simulink model "Ghost_f4"  (Simulink 8.1)
settings: Solver=ode1  StartTime=0.0  StopTime=inf  FixedStep=Ts  MaxStep=1e-3  RelTol=1e-3
PostLoadFcn:
  | NREL_Mode=3; Ghost_init;
InitFcn:
  | NREL_Mode=3; Ghost_init;
undefined symbols (not defined in the file): F4, Left, Stim, Ts, type, V
libraries: simulink x44, relay_modbus_lib x12, rtio_generic_modbus x6, rtlab x5, cables_lib x3, PHIL_lib x2, breaker_lib x2, power_quality_lib x2, artemis x1, rtio_opalrt_ml605ex1 x1, ssn_lib x1, controllable_grid_lib x1
(part 2 of 2)

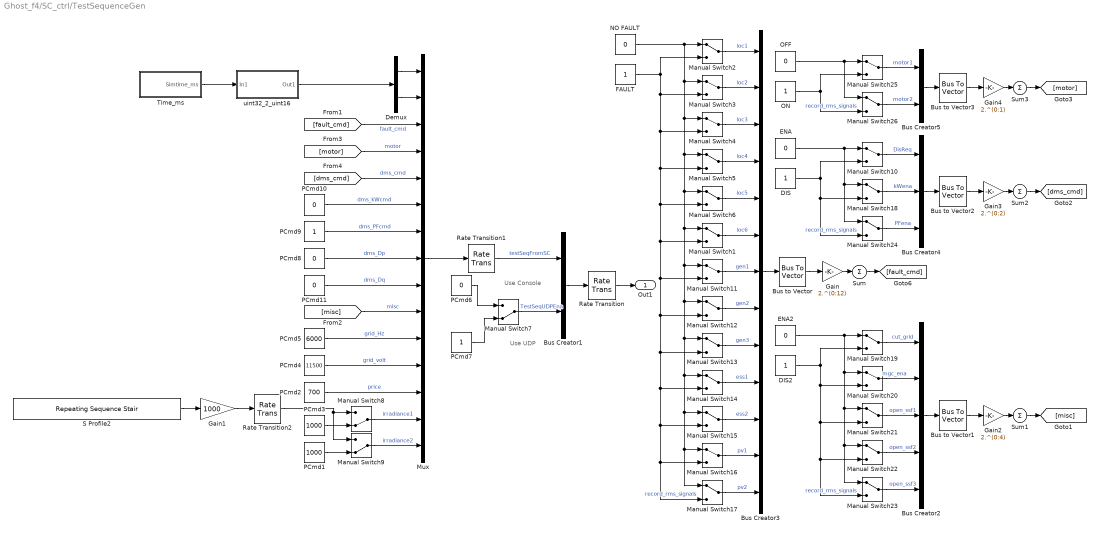
== system Ghost_f4/SC_ctrl/TestSequenceGen ==
  note: Use Console
  note: Use UDP
  Bus Creator1 : BusCreator  Inputs=2
  Bus Creator2 : BusCreator  Inputs=5
  Bus Creator3 : BusCreator  Inputs=13
  Bus Creator4 : BusCreator  Inputs=3
  Bus Creator5 : BusCreator  Inputs=2
  Bus to Vector{,1..3} (4 alike) : BusToVector
  DIS : Constant
  DIS2 : Constant
  Demux : Demux  Outputs=2
  ENA : Constant  Value=0
  ENA2 : Constant  Value=0
  FAULT : Constant
  Gain : Gain  Gain=2.^(0:12)
  Gain1 : Gain  Gain=1000
  Gain2 : Gain  Gain=2.^(0:4)
  Gain3 : Gain  Gain=2.^(0:2)
  Gain4 : Gain  Gain=2.^(0:1)
  Manual Switch{1..6,10..26} (23 alike) : ManualSwitch
  Manual Switch7 : ManualSwitch  CurrentSetting=0
  Manual Switch8 : ManualSwitch  CurrentSetting=0
  Manual Switch9 : ManualSwitch  CurrentSetting=0
  Mux : Mux  Inputs=15
  NO FAULT : Constant  Value=0
  OFF : Constant  Value=0
  ON : Constant
  PCmd1 : Constant  Value=1000
  PCmd10 : Constant  Value=0
  PCmd11 : Constant  Value=0
  PCmd2 : Constant  Value=700
  PCmd3 : Constant  Value=1000
  PCmd4 : Constant  Value=11500
  PCmd5 : Constant  Value=6000
  PCmd6 : Constant  Value=0  SampleTime=[Stim.Ts Ts]
  PCmd7 : Constant
  PCmd8 : Constant  Value=0
  PCmd9 : Constant
  Rate Transition : RateTransition  Deterministic=off
  Rate Transition1 : RateTransition  Deterministic=off  OutPortSampleTime=1e-2
  Rate Transition2 : RateTransition  Deterministic=off  OutPortSampleTime=1e-2
  S Profile2 : simulink/Sources/Repeating Sequence Stair  OutValues=Stim.PV2.Irradiance  tsamp=[Stim.Ts Ts]  OutMin=[]  OutMax=[]  OutDataTypeStr=Inherit: Inherit via back propagation  OutDataType=fixdt(0,8)  ConRadixGroup=Best Precision: Vector-wise  OutScaling=2^-12
  Sum{,1..3} (4 alike) : Sum  Inputs=+
  Time_ms : Subsystem
  uint32_2_uint16 : Subsystem
      mask Display: disp('uint32_2_uint16');
  Out1 : Outport
  wires:
  Manual Switch4/1 -> Bus Creator3/3  "loc3"
  Manual Switch5/1 -> Bus Creator3/4  "loc4"
  [fault_cmd] -> Mux/3  "fault_cmd"
  Bus Creator3/1 -> Bus to Vector/1
  Manual Switch2/1 -> Bus Creator3/1  "loc1"
  Manual Switch6/1 -> Bus Creator3/5  "loc5"
  Manual Switch3/1 -> Bus Creator3/2  "loc2"
  Manual Switch1/1 -> Bus Creator3/6  "loc6"
  Manual Switch13/1 -> Bus Creator3/9  "gen3"
  Manual Switch14/1 -> Bus Creator3/10  "ess1"
  Manual Switch11/1 -> Bus Creator3/7  "gen1"
  Manual Switch15/1 -> Bus Creator3/11  "ess2"
  Manual Switch12/1 -> Bus Creator3/8  "gen2"
  FAULT/1 -> Manual Switch2/2, Manual Switch1/2, Manual Switch12/2, Manual Switch13/2, Manual Switch14/2, Manual Switch17/2, Manual Switch16/2, Manual Switch15/2, Manual Switch11/2, Manual Switch6/2, Manual Switch5/2, Manual Switch4/2, Manual Switch3/2  "record_rms_signals"
  NO FAULT/1 -> Manual Switch12/1, Manual Switch13/1, Manual Switch14/1, Manual Switch15/1, Manual Switch17/1, Manual Switch16/1, Manual Switch11/1, Manual Switch1/1, Manual Switch6/1, Manual Switch5/1, Manual Switch4/1, Manual Switch3/1, Manual Switch2/1
  Manual Switch16/1 -> Bus Creator3/12  "pv1"
  Manual Switch17/1 -> Bus Creator3/13  "pv2"
  Bus to Vector/1 -> Gain/1
  Gain/1 -> Sum/1
  Sum/1 -> [fault_cmd]
  Mux/1 -> Rate Transition1/1
  Bus Creator1/1 -> Rate Transition/1
  Manual Switch7/1 -> Bus Creator1/2  "TestSeqUDPEna"
  PCmd6/1 -> Manual Switch7/1
  PCmd7/1 -> Manual Switch7/2
  Rate Transition/1 -> Out1/1
  PCmd3/1 -> Manual Switch8/2
  Manual Switch9/1 -> Mux/15  "irradiance2"
  PCmd1/1 -> Manual Switch9/2
  Manual Switch8/1 -> Mux/14  "irradiance1"
  PCmd2/1 -> Mux/13  "price"
  Gain1/1 -> Rate Transition2/1
  Time_ms/1(Simtime_ms) -> uint32_2_uint16/1(In1)
  Demux/1 -> Mux/1
  Demux/2 -> Mux/2
  PCmd4/1 -> Mux/12  "grid_volt"
  PCmd5/1 -> Mux/11  "grid_Hz"
  [misc] -> Mux/10  "misc"
  [motor] -> Mux/4  "motor"
  [dms_cmd] -> Mux/5  "dms_cmd"
  PCmd8/1 -> Mux/8  "dms_Dp"
  PCmd9/1 -> Mux/7  "dms_PFcmd"
  PCmd10/1 -> Mux/6  "dms_kWcmd"
  PCmd11/1 -> Mux/9  "dms_Dq"
  Manual Switch21/1 -> Bus Creator2/3  "open_ssf1"
  Manual Switch22/1 -> Bus Creator2/4  "open_ssf2"
  Bus Creator2/1 -> Bus to Vector1/1
  Manual Switch19/1 -> Bus Creator2/1  "cut_grid"
  Manual Switch23/1 -> Bus Creator2/5  "open_ssf3"
  Manual Switch20/1 -> Bus Creator2/2  "mgc_ena"
  DIS2/1 -> Manual Switch20/2, Manual Switch21/2, Manual Switch22/2, Manual Switch23/2, Manual Switch19/2  "record_rms_signals"
  ENA2/1 -> Manual Switch19/1, Manual Switch20/1, Manual Switch21/1, Manual Switch22/1, Manual Switch23/1
  Bus to Vector1/1 -> Gain2/1
  Gain2/1 -> Sum1/1
  Sum1/1 -> [misc]
  Manual Switch24/1 -> Bus Creator4/3  "PFena"
  Bus Creator4/1 -> Bus to Vector2/1
  Manual Switch10/1 -> Bus Creator4/1  "DisReq"
  Manual Switch18/1 -> Bus Creator4/2  "kWena"
  DIS/1 -> Manual Switch10/2, Manual Switch24/2, Manual Switch18/2  "record_rms_signals"
  ENA/1 -> Manual Switch24/1, Manual Switch18/1, Manual Switch10/1
  Bus to Vector2/1 -> Gain3/1
  Gain3/1 -> Sum2/1
  Sum2/1 -> [dms_cmd]
  Bus Creator5/1 -> Bus to Vector3/1
  Manual Switch25/1 -> Bus Creator5/1  "motor1"
  Manual Switch26/1 -> Bus Creator5/2  "motor2"
  ON/1 -> Manual Switch26/2, Manual Switch25/2  "record_rms_signals"
  OFF/1 -> Manual Switch25/1, Manual Switch26/1
  Bus to Vector3/1 -> Gain4/1
  Gain4/1 -> Sum3/1
  Sum3/1 -> [motor]
  S Profile2/1 -> Gain1/1
  uint32_2_uint16/1(Out1) -> Demux/1
  Rate Transition1/1 -> Bus Creator1/1  "testSeqFromSC"
  Rate Transition2/1 -> Manual Switch9/1, Manual Switch8/1

== system Ghost_f4/SS_F4_RELAY_HOUSING/BESS_data ==
  note: 0 .... 10000
      | 0 ... 100%
  Bus Selector1 : BusSelector  OutputSignals=Battery.SoC
  Bus Selector9 : BusSelector  OutputSignals=ESS_DATA
  Constant2 : Constant  Value=0
  Mux : Mux  Inputs=2
  Scale_SoC : Gain  Gain=100
  Out1 : Outport
  wires:
  Scale_SoC/1 -> Out1/1
  [F4_MS_IN] -> Bus Selector9/1
  Bus Selector9/1 -> Bus Selector1/1  "<ESS_DATA>"
  Bus Selector1/1 -> Mux/2  "<SoC>"
  Constant2/1 -> Mux/1
  Mux/1 -> Scale_SoC/1

== system Ghost_f4/SS_F4_RELAY_HOUSING/DieselData ==
  Bus Selector : BusSelector  OutputSignals=GEN3_DATA.gen.gal_per_hr,GEN3_DATA.cb.relay_out.m.Vpu
  Constant1 : Constant  Value=0
  Constant4 : Constant  Value=0
  Mux : Mux
  scale_diesel1 : Gain  Gain=100
  scale_diesel2 : Gain  Gain=100
  Out2 : Outport
  wires:
  [F4_MS_IN] -> Bus Selector/1
  Bus Selector/1 -> scale_diesel1/1  "<gal_per_hr>"
  scale_diesel1/1 -> Mux/2
  Constant4/1 -> Mux/1
  Mux/1 -> Out2/1
  scale_diesel2/1 -> Mux/4
  Bus Selector/2 -> scale_diesel2/1  "<Vpu>"
  Constant1/1 -> Mux/3

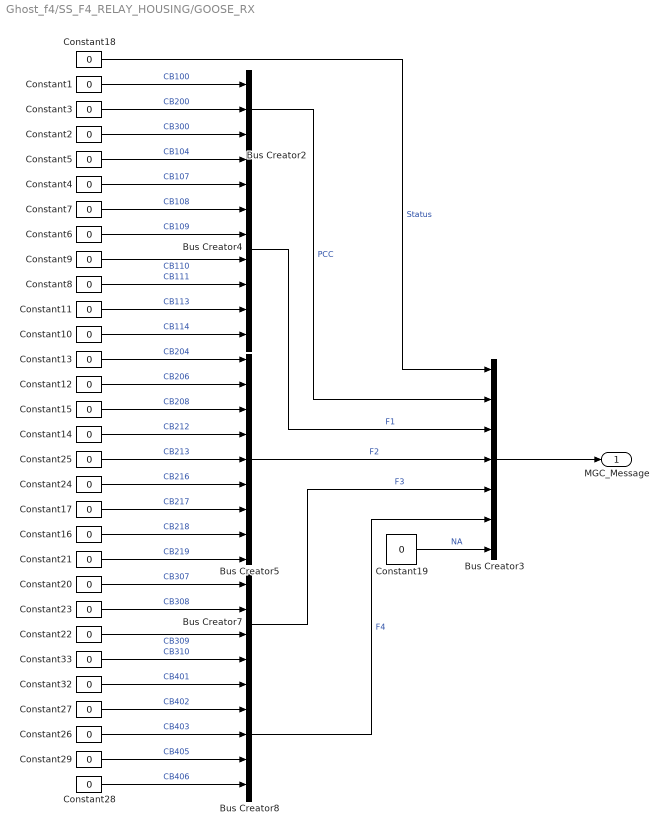
== system Ghost_f4/SS_F4_RELAY_HOUSING/GOOSE_RX  ==
  Bus Creator2 : BusCreator  Inputs=3
  Bus Creator3 : BusCreator  Inputs=7
  Bus Creator4 : BusCreator  Inputs=8
  Bus Creator5 : BusCreator  Inputs=9
  Bus Creator7 : BusCreator
  Bus Creator8 : BusCreator  Inputs=5
  Constant{1..29,32..33} (31 alike) : Constant  Value=0
  MGC_Message : Outport
  wires:
  Constant18/1 -> Bus Creator3/1  "Status"
  Bus Creator3/1 -> MGC_Message/1
  Constant1/1 -> Bus Creator2/1  "CB100"
  Constant3/1 -> Bus Creator2/2  "CB200"
  Constant2/1 -> Bus Creator2/3  "CB300"
  Bus Creator2/1 -> Bus Creator3/2  "PCC"
  Constant7/1 -> Bus Creator4/3  "CB108"
  Constant6/1 -> Bus Creator4/4  "CB109"
  Constant4/1 -> Bus Creator4/2  "CB107"
  Constant9/1 -> Bus Creator4/5  "CB110"
  Constant5/1 -> Bus Creator4/1  "CB104"
  Constant8/1 -> Bus Creator4/6  "CB111"
  Constant11/1 -> Bus Creator4/7  "CB113"
  Constant10/1 -> Bus Creator4/8  "CB114"
  Bus Creator4/1 -> Bus Creator3/3  "F1"
  Constant21/1 -> Bus Creator5/9  "CB219"
  Constant24/1 -> Bus Creator5/6  "CB216"
  Constant17/1 -> Bus Creator5/7  "CB217"
  Constant25/1 -> Bus Creator5/5  "CB213"
  Constant16/1 -> Bus Creator5/8  "CB218"
  Constant15/1 -> Bus Creator5/3  "CB208"
  Constant13/1 -> Bus Creator5/1  "CB204"
  Constant14/1 -> Bus Creator5/4  "CB212"
  Constant12/1 -> Bus Creator5/2  "CB206"
  Bus Creator5/1 -> Bus Creator3/4  "F2"
  Bus Creator8/1 -> Bus Creator3/6  "F4"
  Constant28/1 -> Bus Creator8/5  "CB406"
  Constant26/1 -> Bus Creator8/3  "CB403"
  Bus Creator7/1 -> Bus Creator3/5  "F3"
  Constant33/1 -> Bus Creator7/4  "CB310"
  Constant22/1 -> Bus Creator7/3  "CB309"
  Constant23/1 -> Bus Creator7/2  "CB308"
  Constant20/1 -> Bus Creator7/1  "CB307"
  Constant19/1 -> Bus Creator3/7  "NA"
  Constant29/1 -> Bus Creator8/4  "CB405"
  Constant27/1 -> Bus Creator8/2  "CB402"
  Constant32/1 -> Bus Creator8/1  "CB401"

== system Ghost_f4/SS_F4_RELAY_HOUSING/MGC_controller ==
  Bus Selector1 : BusSelector  OutputSignals=GEN3_DATA,ESS_DATA,PV_DATA
  Bus Selector2 : BusSelector  OutputSignals=ctrl.raw
  Bus Selector3 : BusSelector  OutputSignals=raw
  Bus Selector4 : BusSelector  OutputSignals=raw
  Bus Selector5 : BusSelector  OutputSignals=F4_CB_CTRL  OutputAsBus=on
  Bus to Vector : BusToVector
  Constant : Constant  Value=zeros(1,14)
  Constant1 : Constant  Value=zeros(1,19)
  Constant2 : Constant  Value=zeros(1,10)
  Constant3 : Constant  Value=zeros(1,3)
  Constant{4..7} (4 alike) : Constant  Value=zeros(1,8)
  Vector Concatenate : Concatenate  NumInputs=12
  MGC_controller : Outport
  wires:
  Bus Selector4/1 -> Vector Concatenate/12  "<raw>"
  Constant7/1 -> Vector Concatenate/9
  Constant6/1 -> Vector Concatenate/8
  Constant5/1 -> Vector Concatenate/7
  Constant4/1 -> Vector Concatenate/6
  Bus Selector2/1 -> Vector Concatenate/10  "<raw>"
  Bus Selector3/1 -> Vector Concatenate/11  "<raw>"
  Bus Selector1/3 -> Bus Selector4/1  "<PV_DATA>"
  Bus Selector1/2 -> Bus Selector3/1  "<ESS_DATA>"
  Bus Selector1/1 -> Bus Selector2/1  "<GEN3_DATA>"
  [F4_MS_IN] -> Bus Selector1/1
  Constant2/1 -> Vector Concatenate/3
  Constant1/1 -> Vector Concatenate/2
  Constant/1 -> Vector Concatenate/1
  Constant3/1 -> Vector Concatenate/5
  Vector Concatenate/1 -> MGC_controller/1
  Bus to Vector/1 -> Vector Concatenate/4
  [F4_RELAY_OUT] -> Bus Selector5/1
  Bus Selector5/1 -> Bus to Vector/1

== system Ghost_f4/SS_F4_RELAY_HOUSING/Misc_data ==
  note: Data ordered as:
      | I-P-C
      | kW-VRMSLL
  Bus Creator : BusCreator  Inputs=2
  Constant : Constant  Value=0
  Constant1 : Constant  Value=zeros(1,9)
  Mux8 : Mux  Inputs=2
  Mux9 : Mux  Inputs=2
  VRMSLL : Subsystem
  kW : Subsystem
  scale_load : Gain
  Out1 : Outport
  wires:
  scale_load/1 -> Mux9/1
  [F4_MS_IN] -> Bus Creator/1  "F4"
  Bus Creator/1 -> VRMSLL/1(In1), kW/1(In1)
  Mux8/1 -> scale_load/1
  Constant1/1 -> Mux9/2
  Mux9/1 -> Out1/1
  Constant/1 -> Bus Creator/2  "zero"
  kW/1(Out1) -> Mux8/1
  VRMSLL/1(Out1) -> Mux8/2

== system Ghost_f4/SS_F4_RELAY_HOUSING/Power_quality_data ==
  Rst : Inport
  Bus Selector2 : BusSelector  OutputSignals=F4_CB_1.m.Vpu,F4_CB_2.m.Vpu,F4_CB_5.m.Vpu  OutputAsBus=on
  Bus Selector7 : BusSelector  OutputSignals=F4_CB_1.m.Hz,F4_CB_2.m.Hz,F4_CB_5.m.Hz  OutputAsBus=on
  Bus to Vector : BusToVector
  Bus to Vector3 : BusToVector
  Constant3 : Constant  Value=zeros(1,20)
  Constant4 : Constant  Value=zeros(1,20)
  IEEE1547a_Hz : power_quality_lib/IEEE1547a_Hz
  IEEE1547a_Volt : power_quality_lib/IEEE1547a_Hz
  Mux : Mux  Inputs=2
  Mux2 : Mux  Inputs=2
  Mux3 : Mux  Inputs=2
  Out1 : Outport
  wires:
  Bus to Vector3/1 -> IEEE1547a_Volt/1
  Bus Selector2/1 -> Bus to Vector3/1
  [F4_RELAY_OUT] -> Bus Selector7/1
  [F4_RELAY_OUT] -> Bus Selector2/1
  Constant3/1 -> Mux/1
  Bus to Vector/1 -> IEEE1547a_Hz/1
  Mux/1 -> Mux3/1
  Mux2/1 -> Mux3/2
  IEEE1547a_Volt/1 -> Mux2/2
  Mux3/1 -> Out1/1
  Constant4/1 -> Mux2/1
  Bus Selector7/1 -> Bus to Vector/1
  IEEE1547a_Hz/1 -> Mux/2
  Rst/1 -> IEEE1547a_Volt/2, IEEE1547a_Hz/2

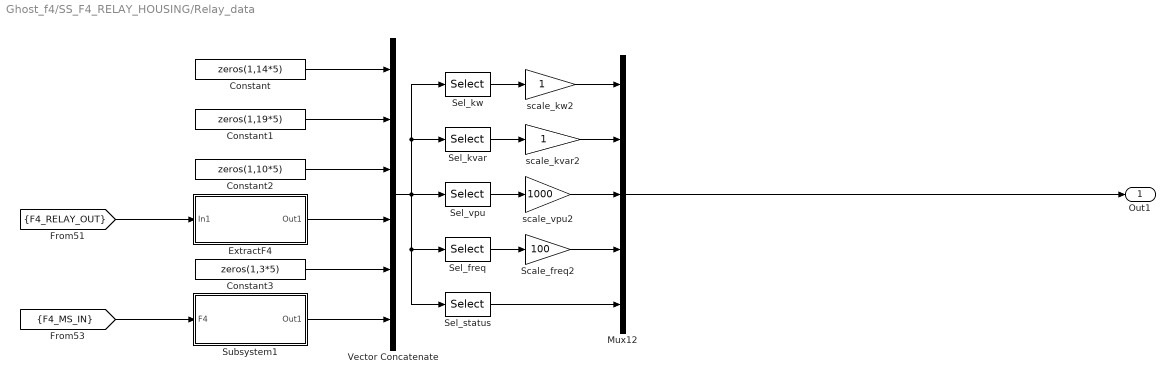
== system Ghost_f4/SS_F4_RELAY_HOUSING/Relay_data ==
  Constant : Constant  Value=zeros(1,14*5)
  Constant1 : Constant  Value=zeros(1,19*5)
  Constant2 : Constant  Value=zeros(1,10*5)
  Constant3 : Constant  Value=zeros(1,3*5)
  ExtractF4 : Subsystem
      mask Display: disp('Generic F4 relays\nID = 44 .. 49')
  Mux12 : Mux  Inputs=5
  Scale_freq2 : Gain  Gain=100
  Sel_freq : Selector  InputPortWidth=59*5  IndexOptions=Index vector (dialog)  Indices=[4:5:59*5]  OutputSizes=1
  Sel_kvar : Selector  InputPortWidth=59*5  IndexOptions=Index vector (dialog)  Indices=[2:5:59*5]  OutputSizes=1
  Sel_kw : Selector  InputPortWidth=59*5  IndexOptions=Index vector (dialog)  Indices=[1:5:59*5]  OutputSizes=1
  Sel_status : Selector  InputPortWidth=59*5  IndexOptions=Index vector (dialog)  Indices=[5:5:59*5]  OutputSizes=1
  Sel_vpu : Selector  InputPortWidth=59*5  IndexOptions=Index vector (dialog)  Indices=[3:5:59*5]  OutputSizes=1
  Subsystem1 : Subsystem
      mask Display: disp('GEN1,ESS1,PV1\nGEN2,GEN3,ESS2,PV1\nID = 53 .. 59')
  Vector Concatenate : Concatenate  NumInputs=6
  scale_kvar2 : Gain
  scale_kw2 : Gain
  scale_vpu2 : Gain  Gain=1000
  Out1 : Outport
  wires:
  [F4_RELAY_OUT] -> ExtractF4/1(In1)
  ExtractF4/1(Out1) -> Vector Concatenate/4
  Constant2/1 -> Vector Concatenate/3
  Constant1/1 -> Vector Concatenate/2
  Constant/1 -> Vector Concatenate/1
  Constant3/1 -> Vector Concatenate/5
  [F4_MS_IN] -> Subsystem1/1(F4)
  Subsystem1/1(Out1) -> Vector Concatenate/6
  Mux12/1 -> Out1/1
  scale_kw2/1 -> Mux12/1
  scale_kvar2/1 -> Mux12/2
  Scale_freq2/1 -> Mux12/4
  scale_vpu2/1 -> Mux12/3
  Sel_kw/1 -> scale_kw2/1
  Sel_status/1 -> Mux12/5
  Sel_freq/1 -> Scale_freq2/1
  Sel_vpu/1 -> scale_vpu2/1
  Sel_kvar/1 -> scale_kvar2/1
  Vector Concatenate/1 -> Sel_status/1, Sel_freq/1, Sel_vpu/1, Sel_kvar/1, Sel_kw/1

== system Ghost_f4/SS_F4_RELAY_HOUSING/Time_ms ==
  Constant4 : Constant  Value=Ts/1e-3
  Sum : Sum  Inputs=++|
  Unit Delay : UnitDelay  SampleTime=-1
  Simtime_ms : Outport
  wires:
  Sum/1 -> Simtime_ms/1, Unit Delay/1
  Constant4/1 -> Sum/2
  Unit Delay/1 -> Sum/1

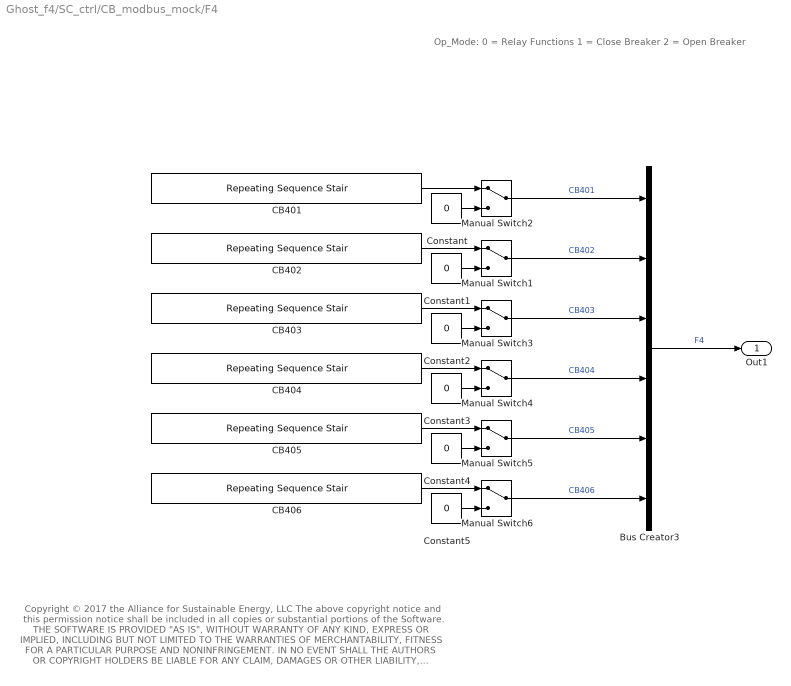
== system Ghost_f4/SC_ctrl/CB_modbus_mock/F4 ==
  note: Op_Mode:
      | 0 = Relay Functions
      | 1 = Close Breaker
      | 2 = Open Breaker
  note: Copyright © 2017 the Alliance for Sustainable Energy, LLC
      |
      | The above copyright notice and this permission notice shall be included in all copies or substantial portions of the Software.
      |
      | THE SOFTWARE IS PROVIDED "AS IS", WITHOUT WARRANTY OF ANY KIND, EXPRESS OR IMPLIED, INCLUDING
      | BUT NOT LIMITED TO THE WARRANTIES OF MERCHANTABILITY, FITNESS FOR A PARTICULAR PURPOSE AND
      | NONINFRINGEMENT. IN NO EVENT SHALL THE AUTHORS OR COPYRIGHT HOLDERS BE LIABLE FOR ANY CLAIM,
      |  DAMAGES OR OTHER LIABILITY, WHETHER IN AN ACTION OF CONTRACT, TORT OR OTHERWISE, ARISING FROM,
      | OUT OF OR IN CONNECTION WITH THE SOFTWARE OR THE USE OR OTHER DEALINGS IN THE SOFTWARE
  Bus Creator3 : BusCreator  Inputs=6
  CB401 : simulink/Sources/Repeating Sequence Stair  OutValues=Stim.CB.CB401  tsamp=[Stim.Ts Ts]  OutMin=[]  OutMax=[]  OutDataTypeStr=Inherit: Inherit via back propagation  OutDataType=fixdt(0,8)  ConRadixGroup=Best Precision: Vector-wise  OutScaling=2^-12
  CB402 : simulink/Sources/Repeating Sequence Stair  OutValues=Stim.CB.CB402  tsamp=[Stim.Ts Ts]  OutMin=[]  OutMax=[]  OutDataTypeStr=Inherit: Inherit via back propagation  OutDataType=fixdt(0,8)  ConRadixGroup=Best Precision: Vector-wise  OutScaling=2^-12
  CB403 : simulink/Sources/Repeating Sequence Stair  OutValues=Stim.CB.CB403  tsamp=[Stim.Ts Ts]  OutMin=[]  OutMax=[]  OutDataTypeStr=Inherit: Inherit via back propagation  OutDataType=fixdt(0,8)  ConRadixGroup=Best Precision: Vector-wise  OutScaling=2^-12
  CB404 : simulink/Sources/Repeating Sequence Stair  OutValues=Stim.CB.CB404  tsamp=[Stim.Ts Ts]  OutMin=[]  OutMax=[]  OutDataTypeStr=Inherit: Inherit via back propagation  OutDataType=fixdt(0,8)  ConRadixGroup=Best Precision: Vector-wise  OutScaling=2^-12
  CB405 : simulink/Sources/Repeating Sequence Stair  OutValues=Stim.CB.CB405  tsamp=[Stim.Ts Ts]  OutMin=[]  OutMax=[]  OutDataTypeStr=Inherit: Inherit via back propagation  OutDataType=fixdt(0,8)  ConRadixGroup=Best Precision: Vector-wise  OutScaling=2^-12
  CB406 : simulink/Sources/Repeating Sequence Stair  OutValues=Stim.CB.CB406  tsamp=[Stim.Ts Ts]  OutMin=[]  OutMax=[]  OutDataTypeStr=Inherit: Inherit via back propagation  OutDataType=fixdt(0,8)  ConRadixGroup=Best Precision: Vector-wise  OutScaling=2^-12
  Constant{,1..5} (6 alike) : Constant  Value=0
  Manual Switch{1..6} (6 alike) : ManualSwitch
  Out1 : Outport
  wires:
  Bus Creator3/1 -> Out1/1  "F4"
  CB401/1 -> Manual Switch2/1
  Constant/1 -> Manual Switch2/2
  Manual Switch2/1 -> Bus Creator3/1  "CB401"
  Manual Switch6/1 -> Bus Creator3/6  "CB406"
  CB402/1 -> Manual Switch1/1
  Manual Switch1/1 -> Bus Creator3/2  "CB402"
  Manual Switch5/1 -> Bus Creator3/5  "CB405"
  Manual Switch3/1 -> Bus Creator3/3  "CB403"
  Manual Switch4/1 -> Bus Creator3/4  "CB404"
  Constant1/1 -> Manual Switch1/2
  CB403/1 -> Manual Switch3/1
  Constant2/1 -> Manual Switch3/2
  CB404/1 -> Manual Switch4/1
  Constant3/1 -> Manual Switch4/2
  CB405/1 -> Manual Switch5/1
  Constant4/1 -> Manual Switch5/2
  CB406/1 -> Manual Switch6/1
  Constant5/1 -> Manual Switch6/2

== system Ghost_f4/SC_ctrl/ESS2 control/Tuning ==
  note: Not applicable
      | for PV
  Bus Creator : BusCreator  Inputs=7
  Constant : Constant  Value=2  SampleTime=[Stim.Ts Ts]
  Constant1 : Constant  Value=0.6e-3  SampleTime=[Stim.Ts Ts]
  Constant10 : Constant  Value=0  SampleTime=[Stim.Ts Ts]
  Constant2 : Constant  Value=180  SampleTime=[Stim.Ts Ts]
  Constant3 : Constant  Value=3200  SampleTime=[Stim.Ts Ts]
  Constant4 : Constant  SampleTime=[Stim.Ts Ts]
  Constant9 : Constant  SampleTime=[Stim.Ts Ts]
  Tuning : Outport
  wires:
  Bus Creator/1 -> Tuning/1
  Constant/1 -> Bus Creator/1  "csi_kp"
  Constant1/1 -> Bus Creator/2  "csi_Ti"
  Constant2/1 -> Bus Creator/3  "pll_kp"
  Constant3/1 -> Bus Creator/4  "pll_ki"
  Constant4/1 -> Bus Creator/5  "vff_ena"
  Constant10/1 -> Bus Creator/7  "batt_soc_rst"
  Constant9/1 -> Bus Creator/6  "batt_cap_div"

== system Ghost_f4/SC_ctrl/PV2 control/Tuning ==
  note: Not applicable
      | for PV
  note: Nominal Insulation = 1000W/m^2
  note: A
      | --------
      | W/m^2
  Bus Creator : BusCreator  Inputs=13
  Constant : Constant  Value=2  SampleTime=[Stim.Ts Ts]
  Constant1 : Constant  Value=0.6e-3  SampleTime=[Stim.Ts Ts]
  Constant10 : Constant  SampleTime=[Stim.Ts Ts]
  Constant12 : Constant  Value=0.2
  Constant13 : Constant  Value=0
  Constant2 : Constant  Value=180  SampleTime=[Stim.Ts Ts]
  Constant3 : Constant  Value=3200  SampleTime=[Stim.Ts Ts]
  Constant4 : Constant  SampleTime=[Stim.Ts Ts]
  Constant5 : Constant  Value=31
  Constant6 : Constant  Value=36
  Constant7 : Constant
  Constant8 : Constant  Value=590
  Constant9 : Constant  SampleTime=[Stim.Ts Ts]
  Tuning : Outport
  wires:
  Constant4/1 -> Bus Creator/5  "vff_ena"
  Constant3/1 -> Bus Creator/4  "pll_ki"
  Constant2/1 -> Bus Creator/3  "pll_kp"
  Constant1/1 -> Bus Creator/2  "csi_Ti"
  Constant/1 -> Bus Creator/1  "csi_kp"
  Bus Creator/1 -> Tuning/1
  Constant6/1 -> Bus Creator/7  "ParallelN"
  Constant5/1 -> Bus Creator/6  "SeriesN"
  Constant7/1 -> Bus Creator/8  "Imin"
  Constant8/1 -> Bus Creator/9  "Vref"
  Constant10/1 -> Bus Creator/11  "batt_soc_rst"
  Constant9/1 -> Bus Creator/10  "batt_cap_div"
  Constant13/1 -> Bus Creator/12  "ConstCurEna"
  Constant12/1 -> Bus Creator/13  "ConstCurGain"

== system Ghost_f4/SC_ctrl/Plots/status_bits_extract ==
  In1 : Inport
  Bias : Bias  Bias=[9:-1:0]*1.1
  Data Type Conversion : DataTypeConversion  OutDataTypeStr=uint16
  Data Type Conversion1 : DataTypeConversion  OutDataTypeStr=double
  Extract Bits1 : simulink/Logic and Bit Operations/Extract Bits  bitsToExtract=Range of bits  numBits=8  bitIdxRange=0  outScalingMode=Treat bit field as an integer
  Extract Bits10 : simulink/Logic and Bit Operations/Extract Bits  bitsToExtract=Range of bits  numBits=8  bitIdxRange=9  outScalingMode=Treat bit field as an integer
  Extract Bits2 : simulink/Logic and Bit Operations/Extract Bits  bitsToExtract=Range of bits  numBits=8  bitIdxRange=1  outScalingMode=Treat bit field as an integer
  Extract Bits3 : simulink/Logic and Bit Operations/Extract Bits  bitsToExtract=Range of bits  numBits=8  bitIdxRange=2  outScalingMode=Treat bit field as an integer
  Extract Bits4 : simulink/Logic and Bit Operations/Extract Bits  bitsToExtract=Range of bits  numBits=8  bitIdxRange=3  outScalingMode=Treat bit field as an integer
  Extract Bits5 : simulink/Logic and Bit Operations/Extract Bits  bitsToExtract=Range of bits  numBits=8  bitIdxRange=4  outScalingMode=Treat bit field as an integer
  Extract Bits6 : simulink/Logic and Bit Operations/Extract Bits  bitsToExtract=Range of bits  numBits=8  bitIdxRange=5  outScalingMode=Treat bit field as an integer
  Extract Bits7 : simulink/Logic and Bit Operations/Extract Bits  bitsToExtract=Range of bits  numBits=8  bitIdxRange=6  outScalingMode=Treat bit field as an integer
  Extract Bits8 : simulink/Logic and Bit Operations/Extract Bits  bitsToExtract=Range of bits  numBits=8  bitIdxRange=7  outScalingMode=Treat bit field as an integer
  Extract Bits9 : simulink/Logic and Bit Operations/Extract Bits  bitsToExtract=Range of bits  numBits=8  bitIdxRange=8  outScalingMode=Treat bit field as an integer
  Mux : Mux  Inputs=10
  Out1 : Outport
  wires:
  Bias/1 -> Out1/1
  Extract Bits5/1 -> Mux/5
  In1/1 -> Data Type Conversion/1
  Extract Bits2/1 -> Mux/2
  Data Type Conversion/1 -> Extract Bits1/1, Extract Bits2/1, Extract Bits3/1, Extract Bits4/1, Extract Bits5/1, Extract Bits8/1, Extract Bits10/1, Extract Bits9/1, Extract Bits7/1, Extract Bits6/1
  Mux/1 -> Data Type Conversion1/1
  Extract Bits1/1 -> Mux/1
  Data Type Conversion1/1 -> Bias/1
  Extract Bits10/1 -> Mux/10
  Extract Bits8/1 -> Mux/8
  Extract Bits9/1 -> Mux/9
  Extract Bits3/1 -> Mux/3
  Extract Bits4/1 -> Mux/4
  Extract Bits7/1 -> Mux/7
  Extract Bits6/1 -> Mux/6

== system Ghost_f4/SC_ctrl/Plots/status_bits_extract1 ==
  In1 : Inport
  Bias : Bias  Bias=[9:-1:0]*1.1
  Data Type Conversion : DataTypeConversion  OutDataTypeStr=uint16
  Data Type Conversion1 : DataTypeConversion  OutDataTypeStr=double
  Extract Bits1 : simulink/Logic and Bit Operations/Extract Bits  bitsToExtract=Range of bits  numBits=8  bitIdxRange=0  outScalingMode=Treat bit field as an integer
  Extract Bits10 : simulink/Logic and Bit Operations/Extract Bits  bitsToExtract=Range of bits  numBits=8  bitIdxRange=9  outScalingMode=Treat bit field as an integer
  Extract Bits2 : simulink/Logic and Bit Operations/Extract Bits  bitsToExtract=Range of bits  numBits=8  bitIdxRange=1  outScalingMode=Treat bit field as an integer
  Extract Bits3 : simulink/Logic and Bit Operations/Extract Bits  bitsToExtract=Range of bits  numBits=8  bitIdxRange=2  outScalingMode=Treat bit field as an integer
  Extract Bits4 : simulink/Logic and Bit Operations/Extract Bits  bitsToExtract=Range of bits  numBits=8  bitIdxRange=3  outScalingMode=Treat bit field as an integer
  Extract Bits5 : simulink/Logic and Bit Operations/Extract Bits  bitsToExtract=Range of bits  numBits=8  bitIdxRange=4  outScalingMode=Treat bit field as an integer
  Extract Bits6 : simulink/Logic and Bit Operations/Extract Bits  bitsToExtract=Range of bits  numBits=8  bitIdxRange=5  outScalingMode=Treat bit field as an integer
  Extract Bits7 : simulink/Logic and Bit Operations/Extract Bits  bitsToExtract=Range of bits  numBits=8  bitIdxRange=6  outScalingMode=Treat bit field as an integer
  Extract Bits8 : simulink/Logic and Bit Operations/Extract Bits  bitsToExtract=Range of bits  numBits=8  bitIdxRange=7  outScalingMode=Treat bit field as an integer
  Extract Bits9 : simulink/Logic and Bit Operations/Extract Bits  bitsToExtract=Range of bits  numBits=8  bitIdxRange=8  outScalingMode=Treat bit field as an integer
  Mux : Mux  Inputs=10
  Out1 : Outport
  wires:
  Extract Bits6/1 -> Mux/6
  Extract Bits7/1 -> Mux/7
  Extract Bits4/1 -> Mux/4
  Extract Bits3/1 -> Mux/3
  Extract Bits9/1 -> Mux/9
  Extract Bits8/1 -> Mux/8
  Extract Bits10/1 -> Mux/10
  Data Type Conversion1/1 -> Bias/1
  Extract Bits1/1 -> Mux/1
  Mux/1 -> Data Type Conversion1/1
  Data Type Conversion/1 -> Extract Bits6/1, Extract Bits7/1, Extract Bits9/1, Extract Bits10/1, Extract Bits8/1, Extract Bits5/1, Extract Bits4/1, Extract Bits3/1, Extract Bits2/1, Extract Bits1/1
  Extract Bits2/1 -> Mux/2
  In1/1 -> Data Type Conversion/1
  Extract Bits5/1 -> Mux/5
  Bias/1 -> Out1/1

== system Ghost_f4/SC_ctrl/TestSequenceGen/Time_ms ==
  Constant4 : Constant  Value=10
  Sum : Sum  Inputs=++|
  Unit Delay : UnitDelay  SampleTime=1e-2
  Simtime_ms : Outport
  wires:
  Unit Delay/1 -> Sum/1
  Constant4/1 -> Sum/2
  Sum/1 -> Unit Delay/1, Simtime_ms/1

== system Ghost_f4/SC_ctrl/TestSequenceGen/uint32_2_uint16 ==
  In1 : Inport
  Data Type Conversion : DataTypeConversion  OutDataTypeStr=uint32
  Data Type Conversion1 : DataTypeConversion  OutDataTypeStr=double
  Data Type Conversion2 : DataTypeConversion  OutDataTypeStr=double
  Extract Bits : simulink/Logic and Bit Operations/Extract Bits  bitsToExtract=Upper half  numBits=8  bitIdxRange=[0 7]  outScalingMode=Treat bit field as an integer
  Extract Bits1 : simulink/Logic and Bit Operations/Extract Bits  bitsToExtract=Lower half  numBits=8  bitIdxRange=[0 7]  outScalingMode=Preserve fixed-point scaling
  Mux : Mux  Inputs=2
  Out1 : Outport
  wires:
  Extract Bits1/1 -> Data Type Conversion2/1
  Data Type Conversion1/1 -> Mux/2
  Data Type Conversion2/1 -> Mux/1
  Data Type Conversion/1 -> Extract Bits/1, Extract Bits1/1
  In1/1 -> Data Type Conversion/1
  Extract Bits/1 -> Data Type Conversion1/1
  Mux/1 -> Out1/1

== system Ghost_f4/SS_F4_RELAY_HOUSING/Misc_data/VRMSLL ==
  In1 : Inport
  Bus Selector29 : BusSelector  OutputSignals=zero,zero,zero,zero,zero,zero,F4.LOAD_DATA.F4_I7.VRMSLL,F4.LOAD_DATA.F4_I8.VRMSLL,zero,zero,zero,zero,zero,zero,F4.LOAD_DATA.F4_P7.VRMSLL,F4.LOAD_DATA.F4_P8.VRMSLL,zero,zero,zero,zero,zero,zero,F4.LOAD_DATA.F4_C7.VRMSLL,F4.LOAD_DATA.F4_C8.VRMSLL,F4.LOAD_DATA.F4_C9.VRMSLL
  Mux : Mux  Inputs=25
  Out1 : Outport
  wires:
  In1/1 -> Bus Selector29/1
  Mux/1 -> Out1/1
  Bus Selector29/1 -> Mux/1  "<zero>"
  Bus Selector29/25 -> Mux/25  "<VRMSLL>"
  Bus Selector29/24 -> Mux/24  "<VRMSLL>"
  Bus Selector29/17 -> Mux/17  "<zero>"
  Bus Selector29/18 -> Mux/18  "<zero>"
  Bus Selector29/19 -> Mux/19  "<zero>"
  Bus Selector29/20 -> Mux/20  "<zero>"
  Bus Selector29/21 -> Mux/21  "<zero>"
  Bus Selector29/22 -> Mux/22  "<zero>"
  Bus Selector29/23 -> Mux/23  "<VRMSLL>"
  Bus Selector29/10 -> Mux/10  "<zero>"
  Bus Selector29/11 -> Mux/11  "<zero>"
  Bus Selector29/12 -> Mux/12  "<zero>"
  Bus Selector29/13 -> Mux/13  "<zero>"
  Bus Selector29/14 -> Mux/14  "<zero>"
  Bus Selector29/15 -> Mux/15  "<VRMSLL>"
  Bus Selector29/16 -> Mux/16  "<VRMSLL>"
  Bus Selector29/3 -> Mux/3  "<zero>"
  Bus Selector29/4 -> Mux/4  "<zero>"
  Bus Selector29/5 -> Mux/5  "<zero>"
  Bus Selector29/6 -> Mux/6  "<zero>"
  Bus Selector29/7 -> Mux/7  "<VRMSLL>"
  Bus Selector29/8 -> Mux/8  "<VRMSLL>"
  Bus Selector29/9 -> Mux/9  "<zero>"
  Bus Selector29/2 -> Mux/2  "<zero>"

== system Ghost_f4/SS_F4_RELAY_HOUSING/Misc_data/kW ==
  In1 : Inport
  Bus Selector28 : BusSelector  OutputSignals=zero,zero,zero,zero,zero,zero,F4.LOAD_DATA.F4_I7.kw,F4.LOAD_DATA.F4_I8.kw,zero,zero,zero,zero,zero,zero,F4.LOAD_DATA.F4_P7.kw,F4.LOAD_DATA.F4_P8.kw,zero,zero,zero,zero,zero,zero,F4.LOAD_DATA.F4_C7.kw,F4.LOAD_DATA.F4_C8.kw,F4.LOAD_DATA.F4_C9.kw
  Mux : Mux  Inputs=25
  Out1 : Outport
  wires:
  In1/1 -> Bus Selector28/1
  Mux/1 -> Out1/1
  Bus Selector28/25 -> Mux/25  "<kw>"
  Bus Selector28/24 -> Mux/24  "<kw>"
  Bus Selector28/23 -> Mux/23  "<kw>"
  Bus Selector28/22 -> Mux/22  "<zero>"
  Bus Selector28/21 -> Mux/21  "<zero>"
  Bus Selector28/20 -> Mux/20  "<zero>"
  Bus Selector28/19 -> Mux/19  "<zero>"
  Bus Selector28/18 -> Mux/18  "<zero>"
  Bus Selector28/17 -> Mux/17  "<zero>"
  Bus Selector28/16 -> Mux/16  "<kw>"
  Bus Selector28/15 -> Mux/15  "<kw>"
  Bus Selector28/14 -> Mux/14  "<zero>"
  Bus Selector28/13 -> Mux/13  "<zero>"
  Bus Selector28/12 -> Mux/12  "<zero>"
  Bus Selector28/11 -> Mux/11  "<zero>"
  Bus Selector28/10 -> Mux/10  "<zero>"
  Bus Selector28/9 -> Mux/9  "<zero>"
  Bus Selector28/8 -> Mux/8  "<kw>"
  Bus Selector28/7 -> Mux/7  "<kw>"
  Bus Selector28/6 -> Mux/6  "<zero>"
  Bus Selector28/5 -> Mux/5  "<zero>"
  Bus Selector28/4 -> Mux/4  "<zero>"
  Bus Selector28/3 -> Mux/3  "<zero>"
  Bus Selector28/2 -> Mux/2  "<zero>"
  Bus Selector28/1 -> Mux/1  "<zero>"

== system Ghost_f4/SS_F4_RELAY_HOUSING/Relay_data/ExtractF4 ==
  In1 : Inport
  Bus Selector47 : BusSelector  OutputSignals=F4_CB_1,F4_CB_2,F4_CB_3,F4_CB_4,F4_CB_5,F4_CB_6
  Bus Selector{48..52,61} (6 alike) : BusSelector  OutputSignals=m.kw,m.kvar,m.Vpu,m.Hz,m.status  OutputAsBus=on
  Mux13 : Mux  Inputs=6
  Out1 : Outport
  wires:
  Bus Selector61/1 -> Mux13/3
  Bus Selector47/5 -> Bus Selector51/1  "<F4_CB_5>"
  Bus Selector49/1 -> Mux13/2
  Bus Selector47/2 -> Bus Selector49/1  "<F4_CB_2>"
  Bus Selector47/3 -> Bus Selector61/1  "<F4_CB_3>"
  Bus Selector47/6 -> Bus Selector52/1  "<F4_CB_6>"
  Bus Selector52/1 -> Mux13/6
  Mux13/1 -> Out1/1
  In1/1 -> Bus Selector47/1
  Bus Selector50/1 -> Mux13/4
  Bus Selector47/1 -> Bus Selector48/1  "<F4_CB_1>"
  Bus Selector47/4 -> Bus Selector50/1  "<F4_CB_4>"
  Bus Selector48/1 -> Mux13/1
  Bus Selector51/1 -> Mux13/5

== system Ghost_f4/SS_F4_RELAY_HOUSING/Relay_data/Subsystem1 ==
  F4 : Inport
  Bus Selector1 : BusSelector  OutputSignals=CB_meas.relay_out.m.kw,CB_meas.relay_out.m.kvar,CB_meas.relay_out.m.Vpu,CB_meas.relay_out.m.Hz,CB_meas.cb_meas.Status  OutputAsBus=on
  Bus Selector10 : BusSelector  OutputSignals=m.kw,m.kvar,m.Vpu,m.Hz,m.status  OutputAsBus=on
  Bus Selector12 : BusSelector  OutputSignals=CB_meas.relay_out.m.kw,CB_meas.relay_out.m.kvar,CB_meas.relay_out.m.Vpu,CB_meas.relay_out.m.Hz,CB_meas.cb_meas.Status  OutputAsBus=on
  Bus Selector3 : BusSelector  OutputSignals=cb.relay_out
  Bus Selector9 : BusSelector  OutputSignals=GEN3_DATA,ESS_DATA,PV_DATA
  Constant{1..4} (4 alike) : Constant  Value=zeros(1,5)
  Mux : Mux  Inputs=7
  Out1 : Outport
  wires:
  Mux/1 -> Out1/1
  Constant2/1 -> Mux/4
  Constant1/1 -> Mux/2
  Constant3/1 -> Mux/1
  Constant4/1 -> Mux/3
  F4/1 -> Bus Selector9/1
  Bus Selector9/1 -> Bus Selector3/1  "<GEN3_DATA>"
  Bus Selector3/1 -> Bus Selector10/1  "<relay_out>"
  Bus Selector10/1 -> Mux/5
  Bus Selector12/1 -> Mux/6
  Bus Selector9/2 -> Bus Selector12/1  "<ESS_DATA>"
  Bus Selector1/1 -> Mux/7
  Bus Selector9/3 -> Bus Selector1/1  "<PV_DATA>"
